simulink model "sim_ssf_sat"  (R2022a)
settings: Solver=VariableStepAuto  StartTime=0.0  StopTime=Tsim  MaxStep=1e-3  RelTol=1e-3
values from neighbouring files (symbols this model uses):
  A = [0.1, - 0.1 ... (first row only)    [aw_polytopic_ct_LTI.m]    (also in aw_sector_ct_LTI.m; sat_polytopic_ct_LTI.m = [-1, 0, 1; sat_sector_ct_LTI.m = [-1, 0, 1)
  B = [5, 0 ... (first row only)    [aw_polytopic_ct_LTI.m]    (also in aw_sector_ct_LTI.m; sat_polytopic_ct_LTI.m = [1; sat_sector_ct_LTI.m = [1)
  C = eye(size(A))    [aw_polytopic_ct_LTI.m]    (also in aw_sector_ct_LTI.m; sat_polytopic_ct_LTI.m; sat_sector_ct_LTI.m)
  D = zeros(size(C,1),size(B,2))    [aw_polytopic_ct_LTI.m]    (also in aw_sector_ct_LTI.m; sat_polytopic_ct_LTI.m; sat_sector_ct_LTI.m)
  K = Y/X    [sat_polytopic_ct_LTI.m]    (also in sat_sector_ct_LTI.m = W/X)
  x0 = [0; 0; 0]    [aw_polytopic_ct_LTI.m]    (also in aw_sector_ct_LTI.m; sat_polytopic_ct_LTI.m = [2; 0.65; 0]; sat_sector_ct_LTI.m = [2; 0.65; 0])
settings Model: Creator=gabriel  LastModifiedBy=gfm

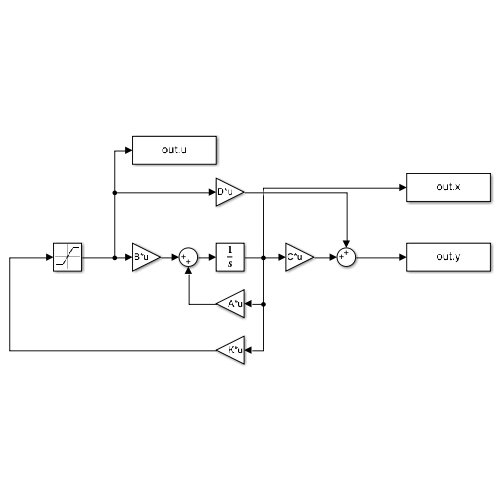
[thumbnail: Simulink's stored preview of the top-level diagram]
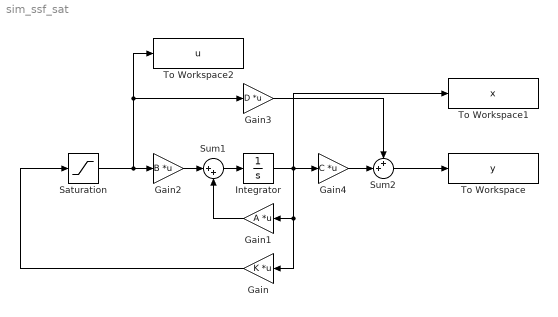
== system sim_ssf_sat ==
  Gain : Gain  Gain=K  Multiplication=Matrix(K*u)
  Gain1 : Gain  Gain=A  Multiplication=Matrix(K*u)
  Gain2 : Gain  Gain=B  Multiplication=Matrix(K*u)
  Gain3 : Gain  Gain=D  Multiplication=Matrix(K*u)
  Gain4 : Gain  Gain=C  Multiplication=Matrix(K*u)
  Integrator : Integrator  InitialCondition=x0
  Saturation : Saturate  UpperLimit=1  LowerLimit=-1
  Sum1 : Sum  Inputs=|++
  Sum2 : Sum  Inputs=++|
  To Workspace : ToWorkspace  VariableName=y  SaveFormat=Structure With Time  SampleTime=-1
  To Workspace1 : ToWorkspace  VariableName=x  SaveFormat=Structure With Time  SampleTime=-1
  To Workspace2 : ToWorkspace  VariableName=u  SaveFormat=Structure With Time  SampleTime=-1
  wires:
  Gain/1 -> Saturation/1
  Integrator/1 -> To Workspace1/1, Gain/1, Gain1/1, Gain4/1
  Gain2/1 -> Sum1/1
  Sum1/1 -> Integrator/1
  Gain1/1 -> Sum1/2
  Gain4/1 -> Sum2/2
  Gain3/1 -> Sum2/1
  Sum2/1 -> To Workspace/1
  Saturation/1 -> Gain2/1, To Workspace2/1, Gain3/1
